simulink model "simulator"  (R2021a)
settings: Solver=ode3  StartTime=0.0  StopTime=5000  FixedStep=1  RelTol=1e-3
InitFcn:
  | clear all
  | clc
  | 
  | %run config_Houston.m
  | run config_Malaga.m
  | 
  | load('PBNsim_buses');
StartFcn:
  | rng('shuffle');
undefined symbols (not defined in the file): entity, initX, instancedAC, m, n, WP, WPabort, WPnext, WPspeed
libraries: AC x23, aerolibactuator x3
(part 1 of 2)
settings Model: OrderedModelArguments=off  Creator=rcasado  LastModifiedBy=usuario
settings SolverCC: AlgebraicLoopSolver=TrustRegion
settings DataIOCC: ReturnWorkspaceOutputs=off
settings DebuggingCC: SFMachineParentedDataDiag=warning  ArithmeticOperatorsInVariantConditions=warning
settings SFSimCC: SimUseLocalCustomCode=off  CustomCodeUndefinedFunction=UseInterfaceOnly
settings RTWCC: RTWUseLocalCustomCode=off
settings CodeAppCC: StateflowObjectComments=on

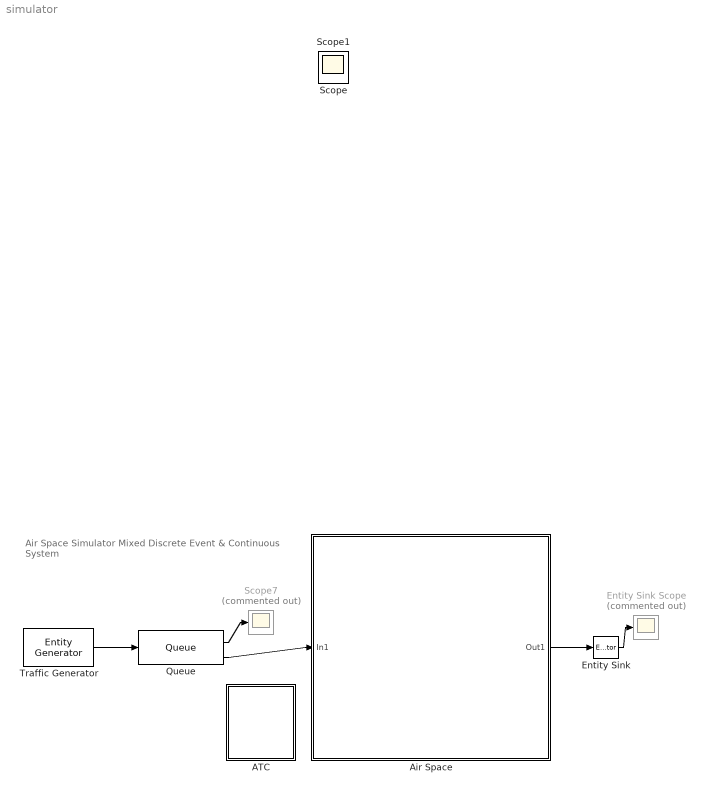
== system simulator ==
  note: Air Space Simulator
      | Mixed Discrete Event & Continuous System
  ATC : Subsystem
      mask Display: image('assets/ATC.svg');
  Air Space : Subsystem
  Entity Sink : EntityTerminator  InputPortMessageModes=m  EntryAction=|  NumberEntitiesArrived=on
      | coder.extrinsic('get_param')
      | currentTime = 0;
      | %currentTime = get_param('simulator18b','SimulationTime');
      | currentTime = get_param(get_param(0,'CurrentSystem'),'SimulationTime');
      | flightTime  = currentTime -entity.startTime;
      | 
      | fprintf('%5.0f: aeronave %3.0f aterriza en %4.0f s\n',...
      |     currentTime,...
      |     entity.flightId,...
      |     flightTime);
      settings: OutputPortMap=o0
  Entity Sink Scope : Scope  Commented=on
  Queue : Queue  InputPortMessageModes=m  OutputPortMessageModes=n,m  Capacity=10  PrioritySource=PriorityAttributeName  BlockedAction=|  NumberEntitiesInBlock=on
      | coder.extrinsic('set_param','gcs');
      | set_param(gcs, 'SimulationCommand', 'stop');
      | 
      | disp('Simulación interrumpida: no hay aviones suficientes para satisfacer la demanda de tráfico aéreo');
      settings: OutputPortMap=o1,o5
  Scope7 : Scope  Commented=on
  Traffic Generator : EntityGenerator  OutputPortMessageModes=m  TimeSource=MATLAB action  Period=120  IntergenerationTimeAction=|  GenerateAction=|  AttributeName=flightId|startTime  AttributeInitialValue=0|0  EntityType=Structured  EntityTypeName=aircraft
      IntergenerationTimeAction=|
      | % Pattern: Repeating Sequence
      | persistent SEQ1;
      | persistent idx1;
      | if isempty(SEQ1)
      |     
      |     % PRUEBAS EN MALAGA: 
      |     SEQ1 = [ 90 90 90 90 90 90 90 90         180        90 ];
      |     
      |     idx1 = 1;
      | end
      | 
      | dt = SEQ1(idx1);
      | 
      | if idx1 == numel(SEQ1)
      |     idx1 = 1;    
      | else
      |     idx1 = idx1 + 1;
      | end
      | 
      | %% para generar un solo avion descomentar lo siguiente
      | % dt = inf
      GenerateAction=|
      | persistent next_flightId;
      | if isempty(next_flightId)
      |     next_flightId = 1;
      | end
      | entity.flightId = next_flightId;
      | next_flightId = next_flightId + 1;
      | 
      | coder.extrinsic('get_param')
      | %entity.startTime = get_param('simulator18b','SimulationTime');
      | entity.startTime = get_param(get_param(0,'CurrentSystem'),'SimulationTime');
      | fprintf('%5.0f: aeronave %3.0f entra en espacio aereo\n',entity.startTime,entity.flightId);
  Scope : Scope
  Scope1 : Scope
  wires:
  Traffic Generator/1 -> Queue/1
  Queue/1 -> Scope7/1
  Entity Sink/1 -> Entity Sink Scope/1
  Queue/2 -> Air Space/1(In1)
  Air Space/1(Out1) -> Entity Sink/1

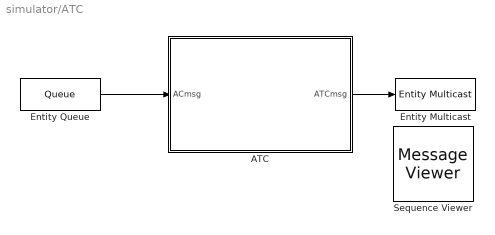
== system simulator/ATC ==
  ATC : Stateflow chart  TreatAsAtomicUnit=on
  Entity Multicast : EntityMulticast  InputPortMessageModes=m  MulticastTag=ATCcomm
  Entity Queue : Queue  OutputPortMessageModes=m  Capacity=100  EntityArrivalSource=Multicast  MulticastTag=ACcomm
  Sequence Viewer : MessageViewer  History=1000
  wires:
  ATC/1(ATCmsg) -> Entity Multicast/1
  Entity Queue/1 -> ATC/1(ACmsg)

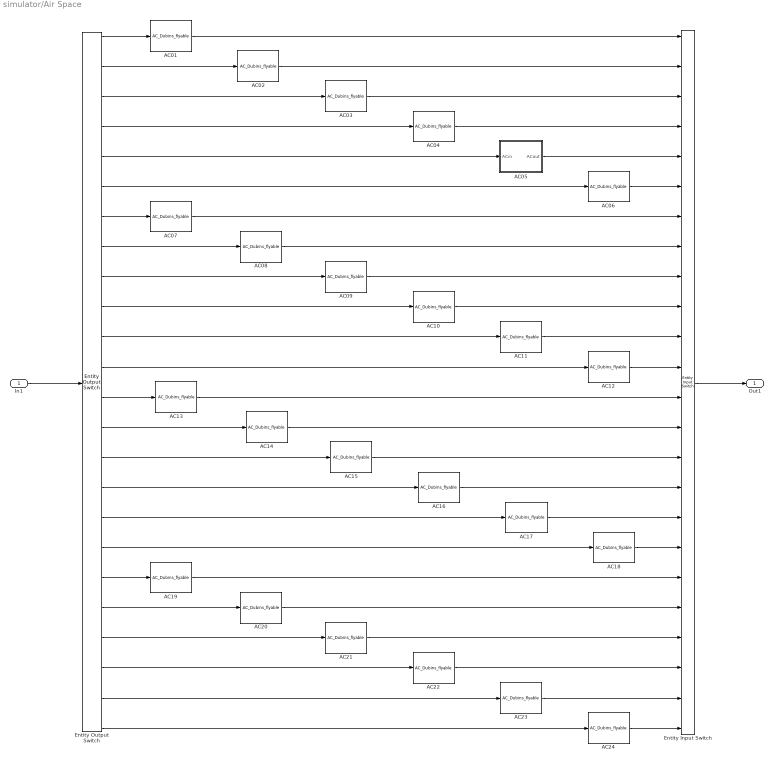
== system simulator/Air Space ==
  In1 : Inport
  AC01 : AC/AC_Dubins_flyable  SystemSampleTime=-1  VariantActivationTime=update diagram  Latency=0  AutoFrameSizeCalculation=off
  AC02 : AC/AC_Dubins_flyable  SystemSampleTime=-1  VariantActivationTime=update diagram  Latency=0  AutoFrameSizeCalculation=off
  AC03 : AC/AC_Dubins_flyable  SystemSampleTime=-1  VariantActivationTime=update diagram  Latency=0  AutoFrameSizeCalculation=off
  AC04 : AC/AC_Dubins_flyable  SystemSampleTime=-1  VariantActivationTime=update diagram  Latency=0  AutoFrameSizeCalculation=off
  AC05 : Subsystem
  AC06 : AC/AC_Dubins_flyable  SystemSampleTime=-1  VariantActivationTime=update diagram  Latency=0  AutoFrameSizeCalculation=off
  AC07 : AC/AC_Dubins_flyable  SystemSampleTime=-1  VariantActivationTime=update diagram  Latency=0  AutoFrameSizeCalculation=off
  AC08 : AC/AC_Dubins_flyable  SystemSampleTime=-1  VariantActivationTime=update diagram  Latency=0  AutoFrameSizeCalculation=off
  AC09 : AC/AC_Dubins_flyable  SystemSampleTime=-1  VariantActivationTime=update diagram  Latency=0  AutoFrameSizeCalculation=off
  AC{10..24} (15 alike) : AC/AC_Dubins_flyable  SystemSampleTime=-1  VariantActivationTime=update diagram  Latency=0  AutoFrameSizeCalculation=off
  Entity Input Switch : EntityInputSwitch  InputPortMessageModes=m,m,m,m,m,m,m,m,m,m,m,m,m,m,m,m,m,m,m,m,m,m,m,m  OutputPortMessageModes=m  NumberInputPorts=24
      settings: InputPortMap=u1,u2,u3,u4,u5,u6,u7,u8,u9,u10,u11,u12,u13,u14,u15,u16,u17,u18,u19,u20,u21,u22,u23,u24
  Entity Output Switch : EntityOutputSwitch  InputPortMessageModes=m  OutputPortMessageModes=m,m,m,m,m,m,m,m,m,m,m,m,m,m,m,m,m,m,m,m,m,m,m,m  NumberOutputPorts=24  SwitchAttributeName=Attribute1
      settings: OutputPortMap=o0,o1,o2,o3,o4,o5,o6,o7,o8,o9,o10,o11,o12,o13,o14,o15,o16,o17,o18,o19,o20,o21,o22,o23
  Out1 : Outport
  wires:
  Entity Output Switch/1 -> AC01/1
  Entity Output Switch/3 -> AC03/1
  Entity Output Switch/4 -> AC04/1
  AC04/1 -> Entity Input Switch/4
  AC02/1 -> Entity Input Switch/2
  AC01/1 -> Entity Input Switch/1
  AC03/1 -> Entity Input Switch/3
  In1/1 -> Entity Output Switch/1
  Entity Input Switch/1 -> Out1/1
  Entity Output Switch/2 -> AC02/1
  Entity Output Switch/5 -> AC05/1(ACin)
  Entity Output Switch/6 -> AC06/1
  Entity Output Switch/8 -> AC08/1
  AC09/1 -> Entity Input Switch/9
  AC07/1 -> Entity Input Switch/7
  Entity Output Switch/9 -> AC09/1
  Entity Output Switch/11 -> AC11/1
  AC10/1 -> Entity Input Switch/10
  Entity Output Switch/12 -> AC12/1
  Entity Output Switch/10 -> AC10/1
  Entity Output Switch/20 -> AC20/1
  AC21/1 -> Entity Input Switch/21
  AC19/1 -> Entity Input Switch/19
  Entity Output Switch/21 -> AC21/1
  Entity Output Switch/23 -> AC23/1
  AC22/1 -> Entity Input Switch/22
  Entity Output Switch/24 -> AC24/1
  Entity Output Switch/22 -> AC22/1
  AC05/1(ACout) -> Entity Input Switch/5
  AC06/1 -> Entity Input Switch/6
  Entity Output Switch/19 -> AC19/1
  AC24/1 -> Entity Input Switch/24
  AC23/1 -> Entity Input Switch/23
  Entity Output Switch/13 -> AC13/1
  Entity Output Switch/14 -> AC14/1
  Entity Output Switch/15 -> AC15/1
  Entity Output Switch/16 -> AC16/1
  Entity Output Switch/17 -> AC17/1
  Entity Output Switch/18 -> AC18/1
  AC18/1 -> Entity Input Switch/18
  AC17/1 -> Entity Input Switch/17
  AC16/1 -> Entity Input Switch/16
  AC15/1 -> Entity Input Switch/15
  AC13/1 -> Entity Input Switch/13
  AC12/1 -> Entity Input Switch/12
  AC11/1 -> Entity Input Switch/11
  Entity Output Switch/7 -> AC07/1
  AC08/1 -> Entity Input Switch/8
  AC14/1 -> Entity Input Switch/14
  AC20/1 -> Entity Input Switch/20

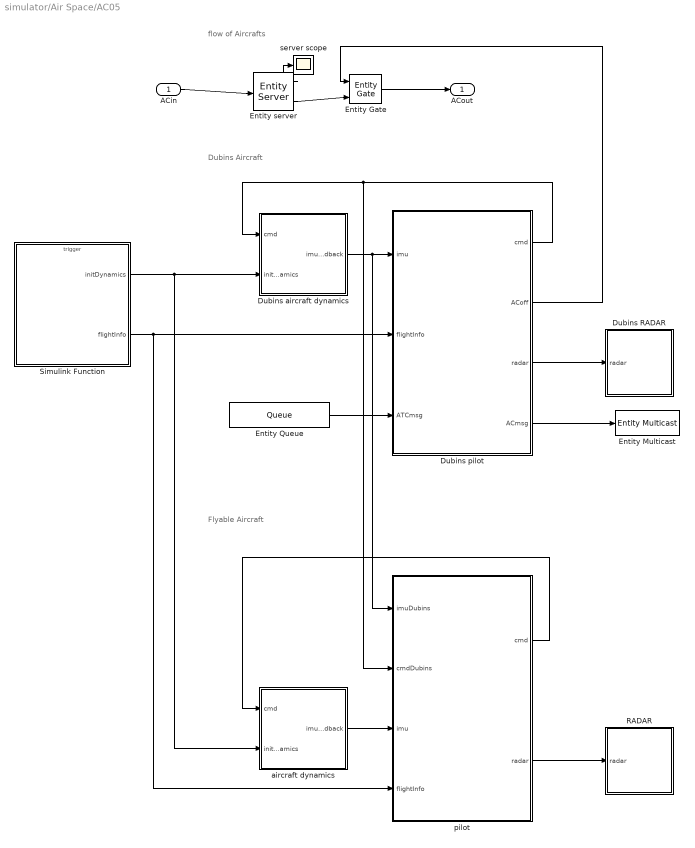
== system simulator/Air Space/AC05 ==
  note: Flyable Aircraft
  note: flow of Aircrafts
  note: Dubins Aircraft
  ACin : Inport
  Dubins RADAR : Subsystem
      mask Display:
      | plot([00 10], [05 05])
      | plot([05 05], [00 10])
      | 
      | plot([01 09 09 01 01], [01 01 09 09 01])
      | plot([03 07 07 03 03], [03 03 07 07 03])
  Dubins aircraft dynamics : Subsystem
      mask Display:
      | patch([50 -50 -50 50], [40 40 -60 -60], [1 1 1])
      | 
      | patch([8 -8 -8 8], [6 6 -6 -6], [0.7 0.7 0.7])
      | 
      | patch([ 8  8  28  28], [0 -2 2 4], [0.5 0.5 0.5])
      | patch([-8 -8 -28 -28], [0 -2 2 4], [0.5 0.5 0.5])
      | 
      | patch([1 0 -1], [6 18 6], [0.5 0.5 0.5])
  Dubins pilot : Stateflow chart  TreatAsAtomicUnit=on
  Entity Gate : EntityGate  InputPortMessageModes=m,m  OutputPortMessageModes=m  OperatingMode=Release gate
  Entity Multicast : EntityMulticast  InputPortMessageModes=m  MulticastTag=ACcomm
  Entity Queue : Queue  OutputPortMessageModes=m  Capacity=100  EntityArrivalSource=Multicast  MulticastTag=ATCcomm
  Entity server : EntityServer  InputPortMessageModes=m  OutputPortMessageModes=n,m  Capacity=1  ServiceTimeValue=10  EntryAction=instancedAC(entity.flightId,true);  ServiceCompleteAction=instancedAC(entity.flightId,false);  NumberEntitiesInBlock=on
      settings: OutputPortMap=o1,o9
  RADAR : Subsystem
      mask Display:
      | plot([00 10], [05 05])
      | plot([05 05], [00 10])
      | 
      | plot([01 09 09 01 01], [01 01 09 09 01])
      | plot([03 07 07 03 03], [03 03 07 07 03])
  Simulink Function : Subsystem  TreatAsAtomicUnit=on
  aircraft dynamics : Subsystem
      mask Display:
      | patch([50 -50 -50 50], [40 40 -60 -60], [1 1 1])
      | 
      | patch([8 -8 -8 8], [6 6 -6 -6], [0.7 0.7 0.7])
      | 
      | patch([ 8  8  28  28], [0 -2 2 4], [0.5 0.5 0.5])
      | patch([-8 -8 -28 -28], [0 -2 2 4], [0.5 0.5 0.5])
      | 
      | patch([1 0 -1], [6 18 6], [0.5 0.5 0.5])
  pilot : Stateflow chart  TreatAsAtomicUnit=on
  server scope : Scope
  ACout : Outport  VectorParamsAs1DForOutWhenUnconnected=off
  wires:
  Entity Queue/1 -> Dubins pilot/3(ATCmsg)
  Entity server/2 -> Entity Gate/2
  Entity Gate/1 -> ACout/1
  Dubins pilot/4(ACmsg) -> Entity Multicast/1
  aircraft dynamics/1(imu_feedback) -> pilot/3(imu)
  Dubins pilot/3(radar) -> Dubins RADAR/1(radar)
  Entity server/1 -> server scope/1
  Dubins pilot/1(cmd) -> Dubins aircraft dynamics/1(cmd), pilot/2(cmdDubins)
  Simulink Function/1(initDynamics) -> Dubins aircraft dynamics/2(initDynamics), aircraft dynamics/2(initDynamics)
  pilot/2(radar) -> RADAR/1(radar)
  Dubins pilot/2(ACoff) -> Entity Gate/1
  pilot/1(cmd) -> aircraft dynamics/1(cmd)
  Dubins aircraft dynamics/1(imu_feedback) -> pilot/1(imuDubins), Dubins pilot/1(imu)
  ACin/1 -> Entity server/1
  Simulink Function/2(flightInfo) -> Dubins pilot/2(flightInfo), pilot/4(flightInfo)

== system simulator/Air Space/AC05/Dubins RADAR ==
  radar : Inport
  RADAR figure : MATLABFcn  StartFcn=|  MATLABFcn=PBNsim_RADAR  OutputDimensions=0  Output1D=off
      | clear functions;
      | clc;
      mask Display: patch([50 -50 -50 50], [40 40 -60 -60], [1 1 1])
  virtual bus : Subsystem
  wires:
  radar/1 -> virtual bus/1(nvbus)
  virtual bus/1(vbus) -> RADAR figure/1

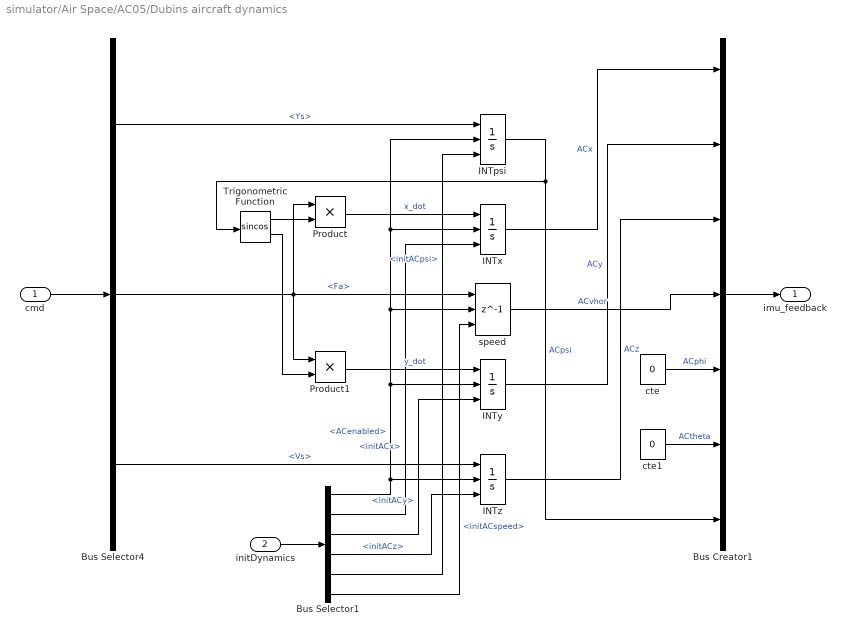
== system simulator/Air Space/AC05/Dubins aircraft dynamics ==
  cmd : Inport
  initDynamics : Inport  Port=2
  Bus Creator1 : BusCreator  Inputs=7  OutDataTypeStr=Bus: bus_IMU
      settings: InheritFromInputs=off
  Bus Selector1 : BusSelector  OutputSignals=ACenabled,initACx,initACy,initACz,initACpsi,initACspeed
  Bus Selector4 : BusSelector  OutputSignals=Ys,Fa,Vs
  INTpsi : Integrator  ExternalReset=rising  InitialConditionSource=external  InitialCondition=initX(3)
  INTx : Integrator  ExternalReset=rising  InitialConditionSource=external  InitialCondition=initX(3)
  INTy : Integrator  ExternalReset=rising  InitialConditionSource=external  InitialCondition=initX(3)
  INTz : Integrator  ExternalReset=rising  InitialConditionSource=external  InitialCondition=initX(3)
  Product : Product
  Product1 : Product
  Trigonometric Function : Trigonometry  Operator=sincos
  cte : Constant  Value=0
  cte1 : Constant  Value=0
  speed : Delay  DelayLength=1  InitialConditionSource=Input port  InitialCondition=convvel(240,'kts','m/s');  ExternalReset=Rising
      settings: InputPortMap=u0,r5,p4
  imu_feedback : Outport  SourceOfInitialOutputValue=Input signal  OutputWhenDisabled=reset  VectorParamsAs1DForOutWhenUnconnected=off
  wires:
  Bus Selector1/6 -> speed/3  "<initACspeed>"
  speed/1 -> Bus Creator1/4  "ACvhor"
  INTpsi/1 -> Trigonometric Function/1, Bus Creator1/7  "ACpsi"
  Bus Selector1/1 -> INTy/2, INTx/2, INTpsi/2, speed/2, INTz/2  "<ACenabled>"
  Bus Selector1/5 -> INTpsi/3  "<initACpsi>"
  Bus Selector1/4 -> INTz/3  "<initACz>"
  Bus Selector1/3 -> INTy/3  "<initACy>"
  Bus Selector1/2 -> INTx/3  "<initACx>"
  initDynamics/1 -> Bus Selector1/1
  Bus Creator1/1 -> imu_feedback/1
  INTy/1 -> Bus Creator1/2  "ACy"
  cte/1 -> Bus Creator1/5  "ACphi"
  INTx/1 -> Bus Creator1/1  "ACx"
  INTz/1 -> Bus Creator1/3  "ACz"
  cte1/1 -> Bus Creator1/6  "ACtheta"
  Bus Selector4/1 -> INTpsi/1  "<Ys>"
  cmd/1 -> Bus Selector4/1
  Bus Selector4/3 -> INTz/1  "<Vs>"
  Trigonometric Function/2 -> Product1/2
  Product/1 -> INTx/1  "x_dot"
  Product1/1 -> INTy/1  "y_dot"
  Trigonometric Function/1 -> Product/2
  Bus Selector4/2 -> Product1/1, speed/1, Product/1  "<Fa>"

== system simulator/Air Space/AC05/RADAR ==
  radar : Inport
  RADAR figure : MATLABFcn  StartFcn=|  MATLABFcn=PBNsim_RADAR  OutputDimensions=0  Output1D=off
      | clear functions;
      | clc;
      mask Display: patch([50 -50 -50 50], [40 40 -60 -60], [1 1 1])
  virtual bus : Subsystem
  wires:
  radar/1 -> virtual bus/1(nvbus)
  virtual bus/1(vbus) -> RADAR figure/1

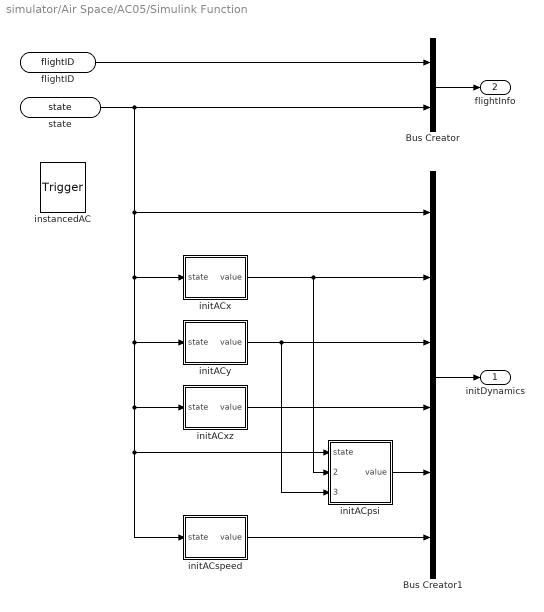
== system simulator/Air Space/AC05/Simulink Function ==
  instancedAC : TriggerPort  TriggerType=function-call  IsSimulinkFunction=on  FunctionName=instancedAC  FunctionVisibility=scoped  VariantControl=Variant
  Bus Creator : BusCreator  Inputs=2  OutDataTypeStr=Bus: bus_ADSB
      settings: InheritFromInputs=off
  Bus Creator1 : BusCreator  Inputs=6  OutDataTypeStr=Bus: bus_initDynamics
      settings: InheritFromInputs=off
  initACpsi : Subsystem
  initACspeed : Subsystem
  initACx : Subsystem
  initACxz : Subsystem
  initACy : Subsystem
  flightID : ArgIn  ArgumentName=flightID
  state : ArgIn  Port=2  OutDataTypeStr=boolean  ArgumentName=state
  initDynamics : Outport  VectorParamsAs1DForOutWhenUnconnected=off
  flightInfo : Outport  Port=2  VectorParamsAs1DForOutWhenUnconnected=off
  wires:
  initACspeed/1(value) -> Bus Creator1/6
  initACpsi/1(value) -> Bus Creator1/5
  initACxz/1(value) -> Bus Creator1/4
  initACy/1(value) -> Bus Creator1/3, initACpsi/3(initACy)
  initACx/1(value) -> Bus Creator1/2, initACpsi/2(initACx)
  Bus Creator1/1 -> initDynamics/1
  flightID/1 -> Bus Creator/1
  Bus Creator/1 -> flightInfo/1
  state/1 -> Bus Creator/2, Bus Creator1/1, initACx/1(state), initACspeed/1(state), initACpsi/1(state), initACxz/1(state), initACy/1(state)

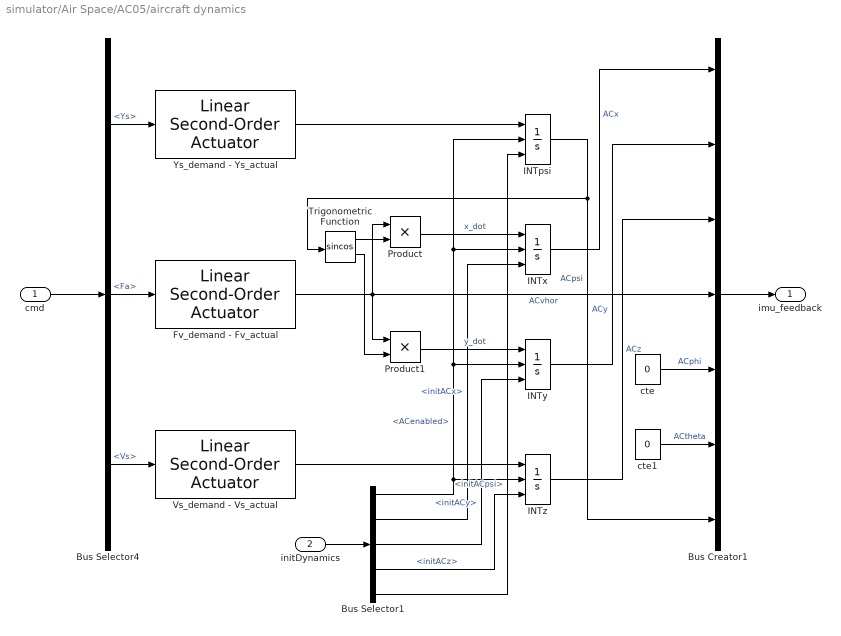
== system simulator/Air Space/AC05/aircraft dynamics ==
  cmd : Inport
  initDynamics : Inport  Port=2
  Bus Creator1 : BusCreator  Inputs=7  OutDataTypeStr=Bus: bus_IMU
      settings: InheritFromInputs=off
  Bus Selector1 : BusSelector  OutputSignals=ACenabled,initACx,initACy,initACz,initACpsi
  Bus Selector4 : BusSelector  OutputSignals=Ys,Fa,Vs
  Fv_demand - Fv_actual : aerolibactuator/Linear Second-Order Actuator  wn_fin=1  z_fin=1  fin_act_0=convvel(240,'kts','m/s');  fin_act_vel=0
      settings: SourceProductBaseCode=AE
  INTpsi : Integrator  ExternalReset=rising  InitialConditionSource=external  InitialCondition=initX(3)
  INTx : Integrator  ExternalReset=rising  InitialConditionSource=external  InitialCondition=initX(3)
  INTy : Integrator  ExternalReset=rising  InitialConditionSource=external  InitialCondition=initX(3)
  INTz : Integrator  ExternalReset=rising  InitialConditionSource=external  InitialCondition=initX(3)
  Product : Product
  Product1 : Product
  Trigonometric Function : Trigonometry  Operator=sincos
  Vs_demand - Vs_actual : aerolibactuator/Linear Second-Order Actuator  wn_fin=1  z_fin=1  fin_act_0=0  fin_act_vel=0
      settings: SourceProductBaseCode=AE
  Ys_demand - Ys_actual : aerolibactuator/Linear Second-Order Actuator  wn_fin=0.8  z_fin=1  fin_act_0=0  fin_act_vel=0
      settings: SourceProductBaseCode=AE
  cte : Constant  Value=0
  cte1 : Constant  Value=0
  imu_feedback : Outport  SourceOfInitialOutputValue=Input signal  OutputWhenDisabled=reset  VectorParamsAs1DForOutWhenUnconnected=off
  wires:
  Ys_demand - Ys_actual/1 -> INTpsi/1
  Vs_demand - Vs_actual/1 -> INTz/1
  INTpsi/1 -> Bus Creator1/7, Trigonometric Function/1  "ACpsi"
  Bus Selector1/1 -> INTy/2, INTx/2, INTpsi/2, INTz/2  "<ACenabled>"
  Bus Selector1/5 -> INTpsi/3  "<initACpsi>"
  Bus Selector1/4 -> INTz/3  "<initACz>"
  Bus Selector1/3 -> INTy/3  "<initACy>"
  Bus Selector1/2 -> INTx/3  "<initACx>"
  initDynamics/1 -> Bus Selector1/1
  Bus Creator1/1 -> imu_feedback/1
  INTy/1 -> Bus Creator1/2  "ACy"
  cte/1 -> Bus Creator1/5  "ACphi"
  INTx/1 -> Bus Creator1/1  "ACx"
  INTz/1 -> Bus Creator1/3  "ACz"
  cte1/1 -> Bus Creator1/6  "ACtheta"
  Bus Selector4/1 -> Ys_demand - Ys_actual/1  "<Ys>"
  cmd/1 -> Bus Selector4/1
  Bus Selector4/3 -> Vs_demand - Vs_actual/1  "<Vs>"
  Trigonometric Function/2 -> Product1/2
  Product/1 -> INTx/1  "x_dot"
  Product1/1 -> INTy/1  "y_dot"
  Trigonometric Function/1 -> Product/2
  Fv_demand - Fv_actual/1 -> Bus Creator1/4, Product1/1, Product/1  "ACvhor"
  Bus Selector4/2 -> Fv_demand - Fv_actual/1  "<Fa>"

== system simulator/Air Space/AC05/Dubins RADAR/virtual bus ==
  nvbus : Inport
  Bus Creator : BusCreator  Inputs=7  OutDataTypeStr=Bus: bus_radar
      settings: InheritFromInputs=off
  Bus Selector4 : BusSelector  OutputSignals=ACid,ACenabled,ACdubins,ACx,ACy,ACz,ACpsi
  vbus : Outport  VectorParamsAs1DForOutWhenUnconnected=off
  wires:
  Bus Selector4/3 -> Bus Creator/3  "<ACdubins>"
  Bus Creator/1 -> vbus/1
  nvbus/1 -> Bus Selector4/1
  Bus Selector4/2 -> Bus Creator/2  "<ACenabled>"
  Bus Selector4/5 -> Bus Creator/5  "<ACy>"
  Bus Selector4/7 -> Bus Creator/7  "<ACpsi>"
  Bus Selector4/6 -> Bus Creator/6  "<ACz>"
  Bus Selector4/4 -> Bus Creator/4  "<ACx>"
  Bus Selector4/1 -> Bus Creator/1  "<ACid>"

== system simulator/Air Space/AC05/RADAR/virtual bus ==
  nvbus : Inport
  Bus Creator : BusCreator  Inputs=7  OutDataTypeStr=Bus: bus_radar
      settings: InheritFromInputs=off
  Bus Selector4 : BusSelector  OutputSignals=ACid,ACenabled,ACdubins,ACx,ACy,ACz,ACpsi
  vbus : Outport  VectorParamsAs1DForOutWhenUnconnected=off
  wires:
  Bus Selector4/3 -> Bus Creator/3  "<ACdubins>"
  Bus Creator/1 -> vbus/1
  nvbus/1 -> Bus Selector4/1
  Bus Selector4/2 -> Bus Creator/2  "<ACenabled>"
  Bus Selector4/5 -> Bus Creator/5  "<ACy>"
  Bus Selector4/7 -> Bus Creator/7  "<ACpsi>"
  Bus Selector4/6 -> Bus Creator/6  "<ACz>"
  Bus Selector4/4 -> Bus Creator/4  "<ACx>"
  Bus Selector4/1 -> Bus Creator/1  "<ACid>"

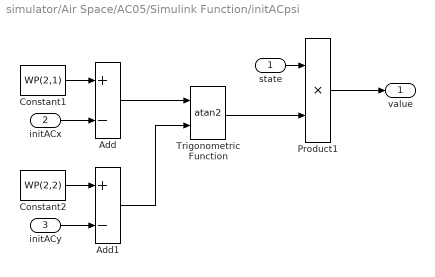
== system simulator/Air Space/AC05/Simulink Function/initACpsi ==
  state : Inport
  initACx : Inport  Port=2
  initACy : Inport  Port=3
  Add : Sum  Inputs=+-
  Add1 : Sum  Inputs=+-
  Constant1 : Constant  Value=WP(2,1)
  Constant2 : Constant  Value=WP(2,2)
  Product1 : Product
  Trigonometric Function : Trigonometry  Operator=atan2
  value : Outport  VectorParamsAs1DForOutWhenUnconnected=off
  wires:
  Product1/1 -> value/1
  Trigonometric Function/1 -> Product1/2
  state/1 -> Product1/1
  Constant1/1 -> Add/1
  initACx/1 -> Add/2
  initACy/1 -> Add1/2
  Constant2/1 -> Add1/1
  Add/1 -> Trigonometric Function/1
  Add1/1 -> Trigonometric Function/2

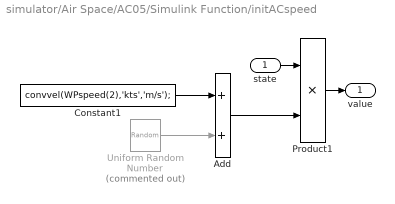
== system simulator/Air Space/AC05/Simulink Function/initACspeed ==
  state : Inport
  Add : Sum
  Constant1 : Constant  Value=convvel(WPspeed(2),'kts','m/s');
  Product1 : Product
  Uniform Random Number : UniformRandomNumber  Commented=on  Minimum=0  Maximum=100  Seed=randi(10000)
  value : Outport  VectorParamsAs1DForOutWhenUnconnected=off
  wires:
  Uniform Random Number/1 -> Add/2
  Product1/1 -> value/1
  state/1 -> Product1/1
  Constant1/1 -> Add/1
  Add/1 -> Product1/2

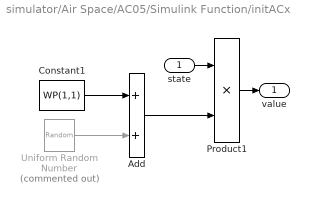
== system simulator/Air Space/AC05/Simulink Function/initACx ==
  state : Inport
  Add : Sum
  Constant1 : Constant  Value=WP(1,1)
  Product1 : Product
  Uniform Random Number : UniformRandomNumber  Commented=on  Minimum=0  Maximum=100  Seed=randi(10000)
  value : Outport  VectorParamsAs1DForOutWhenUnconnected=off
  wires:
  Uniform Random Number/1 -> Add/2
  Product1/1 -> value/1
  state/1 -> Product1/1
  Constant1/1 -> Add/1
  Add/1 -> Product1/2

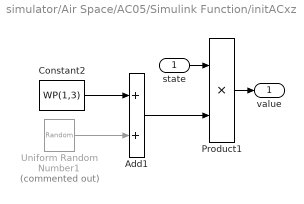
== system simulator/Air Space/AC05/Simulink Function/initACxz ==
  state : Inport
  Add1 : Sum
  Constant2 : Constant  Value=WP(1,3)
  Product1 : Product
  Uniform Random Number1 : UniformRandomNumber  Commented=on  Minimum=0  Maximum=20  Seed=randi(10000)
  value : Outport  VectorParamsAs1DForOutWhenUnconnected=off
  wires:
  Product1/1 -> value/1
  state/1 -> Product1/1
  Constant2/1 -> Add1/1
  Add1/1 -> Product1/2
  Uniform Random Number1/1 -> Add1/2

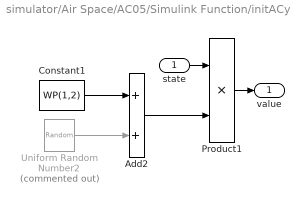
== system simulator/Air Space/AC05/Simulink Function/initACy ==
  state : Inport
  Add2 : Sum
  Constant1 : Constant  Value=WP(1,2)
  Product1 : Product
  Uniform Random Number2 : UniformRandomNumber  Commented=on  Minimum=0  Maximum=100  Seed=randi(10000)
  value : Outport  VectorParamsAs1DForOutWhenUnconnected=off
  wires:
  Product1/1 -> value/1
  state/1 -> Product1/1
  Uniform Random Number2/1 -> Add2/2
  Add2/1 -> Product1/2
  Constant1/1 -> Add2/1

== stateflow chart simulator/Air Space/AC05/Dubins pilot ==
  state NAVIGATOR [parallel]
    settings: executionOrder=1
    state OFF
      entry:
      reset
    state ON
      entry:
      wakeUp
      ACmsgSend
    state FLYING
      entry, during:
      fly
      ACmsgSend
    state SLEEP
      entry:
      sleep
      ACmsgSend
    (default) -> OFF
    OFF -> ON : [flightInfo.ACenabled]
    ON -> FLYING
    SLEEP -> OFF
    FLYING -> SLEEP [order 1] : [landedAC]
    FLYING -> FLYING [order 2] : [abortLanding]
  state COMUNICATIONS [parallel]
    updateRadar
    msgProcess
    settings: executionOrder=2
    state msgProcess [function]
      (default) -> (junction 143)
      (junction 143) -> (junction 138) [order 1] : ATCmsg
      (junction 145) -> (junction 143)
      (junction 143) -> (junction 139) [order 2]
      (junction 138) -> (junction 145) : {ATCmsgProcess}
  data: landed function_output; abort function_output; imu input; cmd output Bus: bus_command; flightInfo input Bus: bus_ADSB; ATCmsg input; ACoff output; radar output Bus: bus_radar; ACmsg output Bus: bus_ACmsg; ACid local double; cWP local; dist local; WP parameter; WPspeed parameter; ACenabled local; ACaborted local
  function reset:
    | function reset
    | 
    | % reseteo estado de la aeronave
    | ACid = 0;
    | ACenabled = 0;
    | ACaborted = 0;
    | 
    | % reseteo movimiento
    | coder.extrinsic('convvel');
    | cmd.Fa = 123.4667; %convvel(cWP(4),'kts','m/s'); %123 m/s
    | cmd.Vs = 0;
    | cmd.Ys = 0;
  function wakeUp:
    | function wakeUp
    | 
    | % inicializo navegación
    | ACid = flightInfo.ACid;
    | ACenabled = 1;
    | cWP = [WP(2,:) WPspeed(2)];
  function landed = landedAC:
    | function landed = landedAC
    | % Concluye si el avion ha terminado de recorrer la pista
    | 
    | landed = false;
    | 
    | if cWP(4) == 50 % la velocidad a 50 solo la tiene el último waypoint
    |     %calculo segmento desde el AC a este WP
    |     s = cWP(1:2)-[imu.ACx imu.ACy];
    |     dist = norm(s);
    |     if dist < 50
    |         landed = true;
    |     end
    | end
  function fly:
    | function fly
    | 
    | % radio de giro
    | r = 2815; % convlength(1.52,'naut mi','m')
    | 
    | %calculo vector AC -> WP actual
    | vec_ac_wp = cWP(1:2) - [imu.ACx imu.ACy];
    | dis_ac_wp = norm(vec_ac_wp);
    | 
    | 
    | %calculo vector AC->dirAC
    | vec_ac_dir = [sin(imu.ACpsi) cos(imu.ACpsi)];
    | 
    | 
    | %determino si el giro es a izquierda o derecha, y el angulo
    | ang_dir_wp = angulo(vec_ac_dir,vec_ac_wp);
    | 
    | 
    | %giramos hacia el lado correcto
    | if ang_dir_wp > 0
    |     % giramos a babor (izquierda)
    |     cmd.Ys = -imu.ACvhor/r;
    |     vec_cc_ac = [sin(imu.ACpsi+pi/2) cos(imu.ACpsi+pi/2)];
    | elseif ang_dir_wp < 0
    |     % giramos a estribor (derecha)
    |     cmd.Ys = +imu.ACvhor/r;
    |     vec_cc_ac = [sin(imu.ACpsi-pi/2) cos(imu.ACpsi-pi/2)];
    | else
    |     % seguimos recto
    |     cmd.Ys = 0;
    |     vec_cc_ac = vec_ac_dir;
    | end
    | 
    | 
    | if ang_dir_wp == 0
    |     dis_hor = dis_ac_wp;
    | else
    | 
    |     %calculo centro de circunferencia de giro
    |     cc = [imu.ACx imu.ACy] - vec_cc_ac * r;
    | 
    |     %compruebo si hay espacio para hacer la curva
    |     vec_cc_wp = cWP(1:2) - cc;
    |     dis_cc_wp = norm(vec_cc_wp);
    |     
    |     if dis_cc_wp < r
    |         % no hay espacio: asumimos recta
    |         dis_hor = dis_ac_wp;
    |     else
    |         %calculo distancia recorrida en linea recta
    |         dis_tc_wp = sqrt(dis_cc_wp^2 - r^2);
    | 
    |         %calculo distancia recorrida en linea curva
    |         ang_cc_tc = atand(r/dis_tc_wp);
    |         ang_tc_wp = 90 - ang_cc_tc;
    |         ang_ac_wp = angulo(vec_cc_ac,vec_cc_wp);
    | 
    |         ang_ac_tc = ang_ac_wp - ang_tc_wp;    
    | 
    |         if sign(ang_dir_wp) == sign(ang_ac_wp)
    |             % tienen el mismo signo: por lo que se gira menos de 1/4 de vuelta
    |             ang_ac_tc = abs(ang_ac_wp) - ang_tc_wp;
    |         else
    |             % tienen signo contrario: por lo que se gira mas de 1/4 de vuelta
    |             ang_ac_tc = 360 - abs(ang_ac_wp) - ang_tc_wp;    
    |         end
    | 
    |         dis_ac_tc = deg2rad(ang_ac_tc) * r;
    | 
    |         %calculo distancia horizontal total a recorrer
    |         dis_hor = dis_ac_tc + dis_tc_wp;         
    |         
    |     end
    |     
    | end
    | 
    | 
    | 
    | vwp    = 0;
    | coder.extrinsic('convvel');
    | vwp    = convvel(cWP(4),'kts','m/s'); %123 m/s
    | 
    | %%
    | % modelo de avion que se adapta a la velocidad del nuevo waypoint 
    | % lo mas rapido posible 
    | cmd.Fa = vwp; %usamos el bus de aceleracion para poner la velocidad deseada
    | 
    | %calculo velocidad vertical
    | dis_vertical = cWP(3) - imu.ACz;
    | tiempo = dis_hor / vwp;
    | cmd.Vs = dis_vertical / tiempo;
    | 
    | 
    | 
    | 
    | 
    | 
    | %%
    | % % modelo de avion que se adapta a la velocidad del nuevo waypoint 
    | % % de manera progresiva en el espacio disponible.
    | % % establece aceleración horizontal al despejar el sistema de ecuaciones:
    | % %    v =  v0 + a * t
    | % %    s = 1/2 * a * t^2
    | % % queda
    | % %    a = (v^2 - v0^2) / 2s
    | % %    t = ( v  -  v0 ) / a
    | % 
    | % % cmd.Fa = (vwp^2 - imu.ACvhor^2) / (2 * dis_hor);
    | % 
    | % 
    | % %calculo velocidad vertical
    | % if cmd.Fa == 0
    | %     % movimiento uniforme
    | %     t = dis_hor / imu.ACvhor;
    | % else
    | %     % movimiento uniformemente acelerado 
    | %     t = (vwp - imu.ACvhor) / cmd.Fa;
    | % end
    | % dist_vertical = cWP(3) - imu.ACz;
    | % cmd.Vs = dist_vertical / t;
    | % 
    | % 
    | % % if imu.ACy < 41000
    | % %     
    | % %     figure
    | % %     hold on
    | % %     grid on
    | % %     axis equal
    | % %     plot(cWP(1),cWP(2),'o')
    | % %     plot(imu.ACx,imu.ACy,'o')
    | % %     plot(cc(1),cc(2),'o')
    | % % end
    | 
    | 
    | 
    | end
    | 
    | 
    | 
    | 
    | 
    | 
    | function a = angulo(V1,V2)
    | % angulo para alcanzar desde V1 a V2
    | % sentido positivo contrario a las agujas del reloj
    | % angulo de salida (-180 +180]
    | 
    |     V1 = V1 / norm(V1);
    |     V2 = V2 / norm(V2);
    | 
    |     prod_esc = V1(1)*V2(1) + V1(2)*V2(2);
    |     if prod_esc > 1
    |         prod_esc = 1;
    |     end
    |     if prod_esc < -1
    |         prod_esc = -1;
    |     end
    |     a1 = acosd(prod_esc);
    | 
    |     prod_vec = V1(1)*V2(2) - V1(2)*V2(1);
    |     a2 = asind(prod_vec);
    |     
    |     a = a1*sign(a2);
    |     
    | end
  function sleep:
    | function sleep
    | 
    | % Desactivamos el avión y dejamos que pase un ciclo 
    | % ara que el RADAR lo elimine
    | ACenabled = 0;
    | 
    | ACoff.data = true;
    | send(ACoff);
  function ACmsgSend:
    | function ACmsgSend
    | ACmsg.data.ACid      = ACid;
    | ACmsg.data.ACenabled = ACenabled;
    | ACmsg.data.ACx       = imu.ACx;
    | ACmsg.data.ACy       = imu.ACy;
    | ACmsg.data.ACz       = imu.ACz;
    | ACmsg.data.ACpsi     = imu.ACpsi;
    | ACmsg.data.ACaborted = ACaborted;
    | send(ACmsg)
  function abort = abortLanding:
    | function abort = abortLanding
    | % Decido si abortar el aterrizaje
    | % 
    | % persistent previously_aborted 
    | % if isempty(previously_aborted)
    | %     previously_aborted = false;
    | % end
    | 
    | abort = false;
    | 
    | if ACaborted
    |     return
    | end
    | 
    | if (ACid == 5) && (imu.ACz < 90) % DA/H: 295 ft (89.9 m)
    |     abort = true;
    |     ACaborted = 1;
    | end
  function updateRadar:
    | function updateRadar
    | 
    | radar.ACid      = ACid;
    | radar.ACenabled = ACenabled;
    | radar.ACdubins  = 1;
    | 
    | radar.ACx       = imu.ACx;
    | radar.ACy       = imu.ACy;
    | radar.ACz       = imu.ACz;
    | radar.ACpsi     = imu.ACpsi;
  function ATCmsgProcess:
    | function ATCmsgProcess
    | 
    | % extraigo informacion del mensaje
    | if ACenabled && ACid == ATCmsg.data.ACid
    |         cWP = [ATCmsg.data.WPx ATCmsg.data.WPy ATCmsg.data.WPz ATCmsg.data.WPspeed];
    | end
    | discard(ATCmsg)
    | 
    | %% Procesamiento del ATC
